simulink model "planmodel_m"  (R2025b)
settings: Solver=ode4  StartTime=0.0  StopTime=200  FixedStep=0.001  RelTol=1e-3
values from neighbouring files (symbols this model uses):
  a0 = 340.294    [plan.m]    (also in plan.mat)
  b_ref = 2.0    (= 2)    [plan.m]    (also in plan.mat)
  c_gear = [0.8e4, 1.4e4, 1.4e4]    [plan.m]    (also in plan.mat = [8000 14000 14000])
  c_lat = [1.4e4, 2.2e4, 2.2e4]    [plan.m]    (also in plan.mat = [14000 22000 22000])
  c_ref = 0.9    [plan.m]    (also in plan.mat)
  c_roll = [0.020, 0.018, 0.018]    [plan.m]    (also in plan.mat = [0.02 0.018 0.018])
  CD0 = 0.045    [plan.m]    (also in plan.mat)
  CL0 = 0.083    [plan.m]    (also in plan.mat)
  CLa = 2.50    (= 2.5)    [plan.m]    (also in plan.mat = 3.8)
  Clb = -0.08    [plan.m]    (also in plan.mat)
  Clda = 0.20    (= 0.2)    [plan.m]    (also in plan.mat = -0.2)
  CLde = 0.25    [plan.m]    (also in plan.mat = 0.28)
  Clp = -0.70    (= -0.7)    [plan.m]    (also in plan.mat)
  CLq = 3.00    (= 3)    [plan.m]    (also in plan.mat = 4.5)
  Clr = 0    [plan.m]    (also in plan.mat = 0.08)
  Cm0 = 0.112    [plan.m]    (also in plan.mat = 0.06)
  Cma = -0.8    [plan.m]    (also in plan.mat)
  Cmde = 0.90    (= 0.9)    [plan.m]    (also in plan.mat = -0.9)
  Cmq = -18.0    (= -18)    [plan.m]    (also in plan.mat)
  Cnb = -0.25    [plan.m]    (also in plan.mat = 0.25)
  Cndr = 0.15    [plan.m]    (also in plan.mat = -0.15)
  Cnp = 0    [plan.m]    (also in plan.mat = -0.04)
  Cnr = -0.45    [plan.m]    (also in plan.mat)
  CSb = -0.8    [plan.m]    (also in plan.mat = -0.7)
  CSdr = 0.18    [plan.m]    (also in plan.mat)
  CSr = 0.15    [plan.m]    (also in plan.mat = 0.12)
  D0 = 800    [plan.m]    (also in plan.mat)
  da_max = 25    [plan.m]    (also in plan.mat)
  da_min = -da_max    (= -25)    [plan.m]    (also in plan.mat)
  de_max = 25    [plan.m]    (also in plan.mat)
  de_min = -de_max    (= -25)    [plan.m]    (also in plan.mat)
  DH = pi / 180    (= 0.0174532925199)    [plan.m]    (also in plan.mat)
  dr_max = 25    [plan.m]    (also in plan.mat)
  dr_min = -dr_max    (= -25)    [plan.m]    (also in plan.mat)
  g = 9.80665    [plan.m]    (also in plan.mat)
  gamma0 = 0.0    (= 0)    [plan.m]
  ground_y = 0.0    (= 0)    [plan.m]
  HD = 180 / pi    (= 57.2957795131)    [plan.m]    (also in plan.mat)
  Ixx = 120.0    (= 120)    [plan.m]    (also in plan.mat)
  Iyy = 480.0    (= 480)    [plan.m]    (also in plan.mat)
  Izz = 520.0    (= 520)    [plan.m]    (also in plan.mat)
  K = 0.080    (= 0.08)    [plan.m]    (also in plan.mat = 0.12)
  K_alpha = 7.67884615385    [plan.mat]
  k_gear = [1.0e5, 3.0e5, 3.0e5]    [plan.m]    (also in plan.mat = [100000 300000 300000])
  k_theta0 = 0.0    (= 0)    [plan.m]
  Kb_to_wy = 10.6510416667    [plan.mat]
  Kn_pitch = 0.117046638908    [plan.mat]
  Kn_to_beta = 0.461367696223    [plan.mat]
  Kw_pitch = -0.524061476442    [plan.mat]
  Kw_to_dr = -1.30612244898    [plan.mat]
  m = 600.0    (= 600)    [plan.m]    (also in plan.mat)
  mu_brake = [0.0, 0.55, 0.55]    [plan.m]    (also in plan.mat = [0 0.55 0.55])
  omigax0 = 0    [plan.m]
  omigay0 = 0    [plan.m]
  omigaz0 = 0    [plan.m]
  psi0 = 0.3/57.3    (= 0.00523560209424)    [plan.m]    (also in plan.mat = 0)
  r_left_b = r_gear_b(:,2)    [plan.m]    (also in plan.mat = [-0.333333333333 -0.8 0.65])
  r_nose_b = r_gear_b(:,1)    [plan.m]    (also in plan.mat = [2 0 0.65])
  r_right_b = r_gear_b(:,3)    [plan.m]    (also in plan.mat = [-0.333333333333 0.8 0.65])
  rho0 = 1.225    [plan.m]    (also in plan.mat)
  S_ref = 1.2    [plan.m]    (also in plan.mat)
  v_eps = 0.20    (= 0.2)    [plan.m]    (also in plan.mat)
  V_min = 1    [plan.m]    (also in plan.mat = 3)
  V_test = 200    [plan.mat]
  Vx0_b = 0.0    (= 0)    [plan.m]
  Vy0_b = 0.0    (= 0)    [plan.m]
  Vz0_b = 0.0    (= 0)    [plan.m]
  W_g = [0; 0; 1]    [plan.m]
  wheel_radius = 0.18    [plan.m]    (also in plan.mat)
  WOW_on = 0.000    (= 0)    [plan.m]    (also in plan.mat)
  Xg0 = 0.0    (= 0)    [plan.m]    (also in plan.mat)
  Yg0 = ground_y + wheel_radius - r_gear_b(2,1) - static_deflection    [plan.m]    (also in plan.mat = 0)
  Zg0 = 1.0    (= 1)    [plan.m]    (also in plan.mat = -0.8215943)
libraries: matrix_library x18, slpidlib x1
(part 2 of 3)

== system planmodel_m/6DOF-MODEL/动力学/体系旋转角速度 ==
  MX : Inport
  MY : Inport  Port=2
  MZ : Inport  Port=3
  Add : Sum
  Add1 : Sum
  Add2 : Sum
  Demux : Demux  Outputs=3
  MATLAB Function : MATLAB Function  TreatAsAtomicUnit=on
  Matrix Multiply1 : Product  Multiplication=Matrix(*)
  Mux : Mux  Inputs=3
  Selector : Selector  InputPortWidth=3  IndexOptions=Index vector (dialog)  Indices=1  OutputSizes=1
  Selector1 : Selector  InputPortWidth=3  IndexOptions=Index vector (dialog)  Indices=2  OutputSizes=1
  Selector2 : Selector  InputPortWidth=3  IndexOptions=Index vector (dialog)  Indices=3  OutputSizes=1
  Subsystem : Subsystem
  Subsystem1 : Subsystem
  Subsystem2 : Subsystem
  wx1 : Outport
  wy1 : Outport  Port=2
  wz1 : Outport  Port=3
  wires:
  Subsystem/1(wx1) -> Subsystem2/2(wx1), Subsystem1/2(wx1), wx1/1
  Subsystem1/1(wy1) -> wy1/1, Subsystem2/3(wy1), Subsystem/3(wy1)
  Subsystem2/1(wz1) -> wz1/1, Subsystem1/3(wz1), Subsystem/2(wz1)
  [M_gear] -> Selector2/1, Selector1/1, Selector/1
  MX/1 -> Add/1
  MY/1 -> Add1/1
  MZ/1 -> Add2/1
  Selector/1 -> Add/2
  Selector2/1 -> Add2/2
  Selector1/1 -> Add1/2
  MATLAB Function/1(R_wind_b) -> Matrix Multiply1/1
  [alpha] -> MATLAB Function/1(alpha)
  [beta] -> MATLAB Function/2(beta)
  Add/1 -> Mux/1
  Add1/1 -> Mux/2
  Add2/1 -> Mux/3
  Mux/1 -> Matrix Multiply1/2
  Demux/1 -> Subsystem/1(MX)
  Matrix Multiply1/1 -> Demux/1
  Demux/2 -> Subsystem1/1(MY)
  Demux/3 -> Subsystem2/1(MZ)

== system planmodel_m/6DOF-MODEL/动力学/姿态角 ==
  wx1 : Inport
  wy1 : Inport  Port=2
  wz1 : Inport  Port=3
  Subsystem : Subsystem
  Subsystem1 : Subsystem
  Subsystem2 : Subsystem
  gamma(eular) : Outport
  theta(eular) : Outport  Port=2
  psi(eular) : Outport  Port=3
  tag scope: gamma_eular=global, psi_eular=global, theta_eular=global
  wires:
  wy1/1 -> Subsystem/2(wy1), Subsystem1/1(wy1), Subsystem2/1(wy1)
  wx1/1 -> Subsystem/1(wx1)
  Subsystem/1(gamma(eular)) -> [gamma_eular], gamma(eular)/1
  wz1/1 -> Subsystem1/2(wz1), Subsystem/3(wz1), Subsystem2/2(wz1)
  Subsystem1/1(theta(eular)) -> [theta_eular], theta(eular)/1
  Subsystem2/1(psi(eular)) -> psi(eular)/1, [psi_eular]

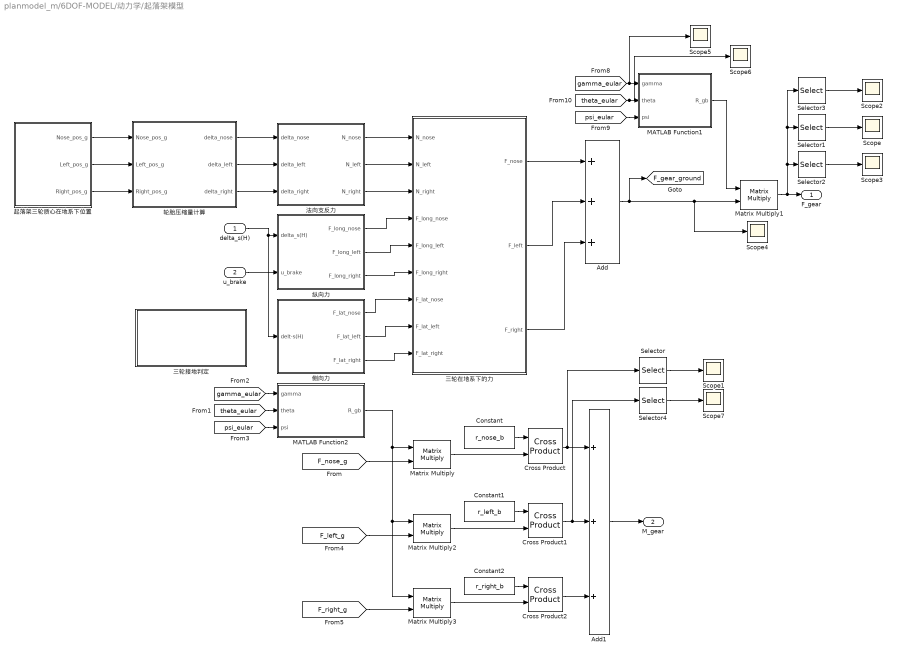
== system planmodel_m/6DOF-MODEL/动力学/起落架模型 ==
  delta_s(H) : Inport
  u_brake : Inport  Port=2
  Add : Sum  Inputs=+++
  Add1 : Sum  Inputs=+++
  Constant : Constant  Value=r_nose_b
  Constant1 : Constant  Value=r_left_b
  Constant2 : Constant  Value=r_right_b
  Cross Product : matrix_library/Cross Product
  Cross Product1 : matrix_library/Cross Product
  Cross Product2 : matrix_library/Cross Product
  MATLAB Function1 : MATLAB Function  TreatAsAtomicUnit=on
  MATLAB Function2 : MATLAB Function  TreatAsAtomicUnit=on
  Matrix Multiply{,1..3} (4 alike) : Product  Multiplication=Matrix(*)
  Scope{,1..7} (8 alike) : Scope
      Scope settings: ActiveDisplayYMinimum=-735.6131  ActiveDisplayYMaximum=6620.5176  DataLoggingVariableName=ScopeData10
      Scope1 settings: ActiveDisplayYMinimum=-1  ActiveDisplayYMaximum=1  DataLoggingVariableName=ScopeData24
      Scope2 settings: ActiveDisplayYMinimum=-144.4872  ActiveDisplayYMaximum=214.9634
      Scope3 settings: ActiveDisplayYMinimum=-1  ActiveDisplayYMaximum=1  DataLoggingVariableName=ScopeData2
      Scope4 settings: ActiveDisplayYMinimum=-856.7234  ActiveDisplayYMaximum=6633.9745  DataLoggingVariableName=ScopeData3
      Scope5 settings: ActiveDisplayYMinimum=1E-13  ActiveDisplayYMaximum=2.6E-13  DataLoggingVariableName=ScopeData4
      Scope6 settings: ActiveDisplayYMinimum=-2E-18  ActiveDisplayYMaximum=3.3E-17  DataLoggingVariableName=ScopeData5
      Scope7 settings: ActiveDisplayYMinimum=-1  ActiveDisplayYMaximum=1  DataLoggingVariableName=ScopeData4
  Selector : Selector  InputPortWidth=3  IndexOptions=Index vector (dialog)  Indices=3  OutputSizes=1
  Selector1 : Selector  InputPortWidth=3  IndexOptions=Index vector (dialog)  Indices=2  OutputSizes=1
  Selector2 : Selector  InputPortWidth=3  IndexOptions=Index vector (dialog)  Indices=3  OutputSizes=1
  Selector3 : Selector  InputPortWidth=3  IndexOptions=Index vector (dialog)  Indices=1  OutputSizes=1
  Selector4 : Selector  InputPortWidth=3  IndexOptions=Index vector (dialog)  Indices=3  OutputSizes=1
  三轮在地系下的力 : Subsystem
  三轮接地判定 : Subsystem
  侧向力 : Subsystem
  法向支反力 : Subsystem
  纵向力 : Subsystem
  起落架三轮质心在地系下位置 : Subsystem
  轮胎压缩量计算 : Subsystem
  F_gear : Outport
  M_gear : Outport  Port=2
  tag scope: F_gear_ground=global
  wires:
  起落架三轮质心在地系下位置/1(Nose_pos_g) -> 轮胎压缩量计算/1(Nose_pos_g)
  起落架三轮质心在地系下位置/2(Left_pos_g) -> 轮胎压缩量计算/2(Left_pos_g)
  起落架三轮质心在地系下位置/3(Right_pos_g) -> 轮胎压缩量计算/3(Right_pos_g)
  轮胎压缩量计算/1(delta_nose) -> 法向支反力/1(delta_nose)
  轮胎压缩量计算/2(delta_left) -> 法向支反力/2(delta_left)
  轮胎压缩量计算/3(delta_right) -> 法向支反力/3(delta_right)
  delta_s(H)/1 -> 侧向力/1(delt-s(H)), 纵向力/1(delta_s(H))
  u_brake/1 -> 纵向力/2(u_brake)
  法向支反力/1(N_nose) -> 三轮在地系下的力/1(N_nose)
  法向支反力/2(N_left) -> 三轮在地系下的力/2(N_left)
  法向支反力/3(N_right) -> 三轮在地系下的力/3(N_right)
  纵向力/1(F_long_nose) -> 三轮在地系下的力/4(F_long_nose)
  纵向力/2(F_long_left) -> 三轮在地系下的力/5(F_long_left)
  纵向力/3(F_long_right) -> 三轮在地系下的力/6(F_long_right)
  侧向力/1(F_lat_nose) -> 三轮在地系下的力/7(F_lat_nose)
  侧向力/2(F_lat_left) -> 三轮在地系下的力/8(F_lat_left)
  侧向力/3(F_lat_right) -> 三轮在地系下的力/9(F_lat_right)
  三轮在地系下的力/1(F_nose) -> Add/1
  三轮在地系下的力/2(F_left) -> Add/2
  三轮在地系下的力/3(F_right) -> Add/3
  Add/1 -> Scope4/1, Matrix Multiply1/2, [F_gear_ground]
  MATLAB Function1/1(R_gb) -> Matrix Multiply1/1
  [gamma_eular] -> Scope5/1, MATLAB Function1/1(gamma)
  Matrix Multiply1/1 -> Selector3/1, Selector1/1, Selector2/1, F_gear/1
  Constant/1 -> Cross Product/1
  Constant1/1 -> Cross Product1/1
  Constant2/1 -> Cross Product2/1
  Cross Product/1 -> Add1/1, Selector/1
  Cross Product1/1 -> Selector4/1, Add1/2
  Cross Product2/1 -> Add1/3
  Add1/1 -> M_gear/1
  [theta_eular] -> Scope6/1, MATLAB Function1/2(theta)
  [psi_eular] -> MATLAB Function1/3(psi)
  [theta_eular] -> MATLAB Function2/2(theta)
  [gamma_eular] -> MATLAB Function2/1(gamma)
  [psi_eular] -> MATLAB Function2/3(psi)
  MATLAB Function2/1(R_gb) -> Matrix Multiply3/1, Matrix Multiply2/1, Matrix Multiply/1
  [F_nose_g] -> Matrix Multiply/2
  [F_right_g] -> Matrix Multiply3/2
  [F_left_g] -> Matrix Multiply2/2
  Matrix Multiply2/1 -> Cross Product1/2
  Matrix Multiply3/1 -> Cross Product2/2
  Matrix Multiply/1 -> Cross Product/2
  Selector1/1 -> Scope/1
  Selector3/1 -> Scope2/1
  Selector2/1 -> Scope3/1
  Selector/1 -> Scope1/1
  Selector4/1 -> Scope7/1

== system planmodel_m/control/俯仰通道控制器/俯仰通道 ==
  nyc : Inport
  ny : Inport  Port=2
  wz : Inport  Port=3
  Constant : Constant
  Div : Product  Inputs=/*
  Gain : Gain
  Gain2 : Gain
  Integrator : Integrator  ExternalReset=either  LimitOutput=on  UpperSaturationLimit=5  LowerSaturationLimit=-5
  Ka : Constant  Value=K_alpha
  Kn : Constant  Value=Kn_pitch
  Kwz : Constant  Value=Kw_pitch
  Pk : Product
  Pn : Product
  Product : Product
  Product1 : Product
  Product2 : Product
  Sat : Saturate  UpperLimit=10  LowerLimit=0.25
  Scope : Scope  NumInputPorts=2
      settings: ActiveDisplayYMinimum=0.47912  ActiveDisplayYMaximum=1.5066
  Sqr : Math  Operator=square
  Sum{,1..3} (4 alike) : Sum  Inputs=|+-
  VRef : Constant  Value=V_test
  伪攻角回路 : Subsystem
  delta_e : Outport
  wires:
  Kn/1 -> Product/1
  VRef/1 -> Div/1
  Integrator/1 -> Sum1/1
  [Vg] -> Div/2
  Pk/1 -> delta_e/1
  nyc/1 -> Sum/1, Scope/1
  ny/1 -> Sum/2, Scope/2
  Div/1 -> Sqr/1
  Sqr/1 -> Sat/1
  Sum/1 -> Product/2
  Product/1 -> Pn/1
  Constant/1 -> Sum3/1
  Sat/1 -> Pn/2, Pk/2
  [no_contact] -> Sum3/2
  Kwz/1 -> Gain2/1
  Pn/1 -> Integrator/1
  Sum3/1 -> Integrator/2
  wz/1 -> 伪攻角回路/1(wz), Sum2/2
  Ka/1 -> Gain/1
  伪攻角回路/1(alpha_c) -> Sum1/2
  Gain/1 -> Product1/1
  Sum1/1 -> Product1/2
  Product1/1 -> Sum2/1
  Gain2/1 -> Product2/1
  Sum2/1 -> Product2/2
  Product2/1 -> Pk/1

== system planmodel_m/control/俯仰通道控制器/抬轮俯仰角控制通道 ==
  theta_cmd(H) : Inport
  Gain1 : Gain
  K_theta : Gain  Gain=1.3
  Sum : Sum  Inputs=|+-
  Sum1 : Sum  Inputs=|+-
  de : Outport
  wires:
  theta_cmd(H)/1 -> Sum/1
  [theta_eular] -> Sum/2
  Sum/1 -> K_theta/1
  K_theta/1 -> Sum1/1
  [wz1] -> Gain1/1
  Gain1/1 -> Sum1/2
  Sum1/1 -> de/1

== system planmodel_m/control/滚转通道控制器/Subsystem ==
  gamma_c : Inport
  wx : Inport  Port=2
  gamma : Inport  Port=3
  Gain1 : Gain  Gain=1/HD
  Integrator : Integrator
  Product : Product
  Product1 : Product
  Product2 : Product
  Scope : Scope  NumInputPorts=2
      settings: ActiveDisplayYMinimum=-0.00046391  ActiveDisplayYMaximum=0.00061315  DataLoggingVariableName=ScopeData2
  Scope1 : Scope
      settings: ActiveDisplayYMinimum=-1  ActiveDisplayYMaximum=1  DataLoggingVariableName=ScopeData47
  Sum : Sum  Inputs=|+-
  Sum1 : Sum  Inputs=|+-
  Sum2 : Sum  Inputs=|++
  kgamma_to_wx : Constant  Value=3
  kigamma_to_wx : Constant
  kwx_to_da : Constant  Value=0.5
  da : Outport
  wires:
  Sum/1 -> Product/2, Product2/2
  Sum1/1 -> Product1/2
  wx/1 -> Sum1/2
  gamma/1 -> Scope/2, Sum/2
  kigamma_to_wx/1 -> Product2/1
  Product2/1 -> Integrator/1
  Product/1 -> Sum2/1
  Sum2/1 -> Sum1/1
  Integrator/1 -> Sum2/2
  Gain1/1 -> Scope/1, Sum/1
  kgamma_to_wx/1 -> Product/1
  kwx_to_da/1 -> Product1/1
  gamma_c/1 -> Gain1/1
  Product1/1 -> Scope1/1, da/1

== system planmodel_m/control/航向通道控制器/偏航通道 ==
  nzc : Inport
  nz : Inport  Port=2
  wy : Inport  Port=3
  Constant1 : Constant
  Constant3 : Constant  Value=0
  Div : Product  Inputs=/*
  Gain : Gain  Gain=-Kn_to_beta
  Gain1 : Gain  Gain=Kb_to_wy
  Gain2 : Gain  Gain=Kw_to_dr
  Gain4 : Gain  Gain=HD
  Integrator : Integrator  ExternalReset=either
  Pk : Product
  Pn : Product
  Sat : Saturate  UpperLimit=10  LowerLimit=0.25
  Saturation1 : Saturate  UpperLimit=0.2*57.3  LowerLimit=-0.2*57.3
  Scope : Scope  NumInputPorts=2
      settings: ActiveDisplayYMinimum=-0.21765504645958114  ActiveDisplayYMaximum=0.42871368847964081
  Scope1 : Scope
      settings: ActiveDisplayYMinimum=-0.34545426181804578  ActiveDisplayYMaximum=0.23208089486151426  DataLoggingVariableName=ScopeData42
  Scope12 : Scope
      settings: ActiveDisplayYMinimum=-1.8487  ActiveDisplayYMaximum=16.1209  DataLoggingVariableName=ScopeData39
  Scope2 : Scope  NumInputPorts=2
      settings: ActiveDisplayYMinimum=-1.0707329995063326  ActiveDisplayYMaximum=0.50557097548372176  DataLoggingVariableName=ScopeData41
  Sqr : Math  Operator=square
  Sum : Sum  Inputs=|+-
  Sum1 : Sum  Inputs=|+-
  Sum2 : Sum  Inputs=|+-
  Switch2 : Switch  Threshold=40  SaturateOnIntegerOverflow=off  InputSameDT=off
  VRef : Constant  Value=V_test
  伪攻角回路 : Subsystem
  delta_r : Outport
  wires:
  nz/1 -> Sum/2, Scope/2
  nzc/1 -> Scope/1, Sum/1
  Constant1/1 -> Switch2/1
  Constant3/1 -> Switch2/3
  [Vg] -> Div/2, Switch2/2
  Gain4/1 -> Scope12/1
  [psi_eular] -> Gain4/1
  wy/1 -> Scope2/2, Sum2/2, 伪攻角回路/1(wy)
  伪攻角回路/1(beta_c) -> Sum1/2
  Sum1/1 -> Gain1/1
  Gain1/1 -> Scope2/1, Sum2/1
  Sum2/1 -> Gain2/1
  Sum/1 -> Gain/1
  Integrator/1 -> Saturation1/1
  Saturation1/1 -> Sum1/1
  Switch2/1 -> Integrator/2
  VRef/1 -> Div/1
  Div/1 -> Sqr/1
  Sqr/1 -> Sat/1
  Sat/1 -> Pn/2, Pk/2
  Gain2/1 -> Pk/1
  Pk/1 -> delta_r/1, Scope1/1
  Gain/1 -> Pn/1
  Pn/1 -> Integrator/1

== system planmodel_m/control/航向通道控制器/地面转向控制 ==
  Z_cmd : Inport
  Gain : Gain  Gain=0.8
  Gain4 : Gain  Gain=HD
  K_z : Constant  Value=0.04
  Product : Product
  Saturation1 : Saturate  UpperLimit=5  LowerLimit=-5
  Scope : Scope  NumInputPorts=2
      settings: ActiveDisplayYMinimum=-14.247959246651458  ActiveDisplayYMaximum=14.936251376866672  DataLoggingVariableName=ScopeData26
  Scope12 : Scope
      settings: ActiveDisplayYMinimum=-16.1569  ActiveDisplayYMaximum=26.4194  DataLoggingVariableName=ScopeData32
  Scope25 : Scope
      settings: ActiveDisplayYMinimum=-11.4126  ActiveDisplayYMaximum=3.1927  DataLoggingVariableName=ScopeData31
  Sum : Sum  Inputs=|+-
  Sum1 : Sum  Inputs=|++
  Transfer Fcn : TransferFcn  Denominator=[0.1 1]
  delta_s(H) : Outport
  wires:
  Z_cmd/1 -> Scope/1, Sum/1
  [Z_positon] -> Scope/2, Sum/2
  K_z/1 -> Product/1
  [delta_s] -> Scope25/1
  [psi_eular] -> Gain/1
  Gain4/1 -> Scope12/1
  [psi_eular] -> Gain4/1
  Gain/1 -> Sum1/2
  Sum/1 -> Saturation1/1
  Product/1 -> Sum1/1
  Saturation1/1 -> Product/2
  Sum1/1 -> Transfer Fcn/1
  Transfer Fcn/1 -> delta_s(H)/1

== system planmodel_m/control/航向通道控制器1/偏航通道 ==
  nzc : Inport
  nz : Inport  Port=2
  wy : Inport  Port=3
  Constant1 : Constant
  Constant3 : Constant  Value=0
  Gain : Gain  Gain=-Kn_to_beta
  Gain1 : Gain  Gain=Kb_to_wy
  Gain2 : Gain  Gain=Kw_to_dr
  Gain4 : Gain  Gain=HD
  Integrator : Integrator  ExternalReset=either
  Saturation1 : Saturate  UpperLimit=0.2*57.3  LowerLimit=-0.2*57.3
  Scope : Scope  NumInputPorts=2
      settings: ActiveDisplayYMinimum=-0.48826  ActiveDisplayYMaximum=1.2494
  Scope1 : Scope
      settings: ActiveDisplayYMinimum=-153.0484  ActiveDisplayYMaximum=1377.4356  DataLoggingVariableName=ScopeData42
  Scope12 : Scope
      settings: ActiveDisplayYMinimum=-151.9167  ActiveDisplayYMaximum=542.4127  DataLoggingVariableName=ScopeData39
  Scope2 : Scope  NumInputPorts=2
      settings: ActiveDisplayYMinimum=-6.2342  ActiveDisplayYMaximum=4.3442  DataLoggingVariableName=ScopeData41
  Sum : Sum  Inputs=|+-
  Sum1 : Sum  Inputs=|+-
  Sum2 : Sum  Inputs=|+-
  Switch2 : Switch  Threshold=40  SaturateOnIntegerOverflow=off  InputSameDT=off
  伪攻角回路 : Subsystem
  delta_r : Outport
  wires:
  nz/1 -> Scope/2, Sum/2
  nzc/1 -> Scope/1, Sum/1
  Constant1/1 -> Switch2/1
  Constant3/1 -> Switch2/3
  [Vg] -> Switch2/2
  Gain4/1 -> Scope12/1
  [psi_eular] -> Gain4/1
  wy/1 -> Scope2/2, Sum2/2, 伪攻角回路/1(wy)
  伪攻角回路/1(beta_c) -> Sum1/2
  Sum1/1 -> Gain1/1
  Gain1/1 -> Scope2/1, Sum2/1
  Sum2/1 -> Gain2/1
  Gain2/1 -> Scope1/1, delta_r/1
  Gain/1 -> Integrator/1
  Sum/1 -> Gain/1
  Integrator/1 -> Saturation1/1
  Saturation1/1 -> Sum1/1
  Switch2/1 -> Integrator/2

== system planmodel_m/control/航向通道控制器1/地面转向控制 ==
  Z_cmd : Inport
  Gain : Gain  Gain=0.8
  Gain4 : Gain  Gain=HD
  K_z : Constant  Value=0.04
  Product : Product
  Saturation1 : Saturate  UpperLimit=5  LowerLimit=-5
  Scope : Scope  NumInputPorts=2
      settings: ActiveDisplayYMinimum=-8.5383  ActiveDisplayYMaximum=8.0262  DataLoggingVariableName=ScopeData26
  Scope12 : Scope
      settings: ActiveDisplayYMinimum=-4.9887  ActiveDisplayYMaximum=24.3498  DataLoggingVariableName=ScopeData32
  Scope25 : Scope
      settings: ActiveDisplayYMinimum=-13.1282  ActiveDisplayYMaximum=3.562  DataLoggingVariableName=ScopeData31
  Sum : Sum  Inputs=|+-
  Sum1 : Sum  Inputs=|++
  delta_s(H) : Outport
  wires:
  Z_cmd/1 -> Scope/1, Sum/1
  [Z_positon] -> Scope/2, Sum/2
  K_z/1 -> Product/1
  [delta_s] -> Scope25/1
  [psi_eular] -> Gain/1
  Gain4/1 -> Scope12/1
  [psi_eular] -> Gain4/1
  Gain/1 -> Sum1/2
  Sum/1 -> Saturation1/1
  Product/1 -> Sum1/1
  Saturation1/1 -> Product/2
  Sum1/1 -> delta_s(H)/1

== system planmodel_m/6DOF-MODEL/AERO-PARAMETER/无量纲化角速率/Subsystem ==
  wy1 : Inport
  Va : Inport  Port=2
  Constant4 : Constant  Value=b_ref
  Divide : Product  Inputs=*/
  Gain : Gain  Gain=2
  Product : Product
  r_hat : Outport
  wires:
  Va/1 -> Gain/1
  wy1/1 -> Product/1
  Constant4/1 -> Product/2
  Product/1 -> Divide/1
  Divide/1 -> r_hat/1
  Gain/1 -> Divide/2

== system planmodel_m/6DOF-MODEL/AERO-PARAMETER/无量纲化角速率/Subsystem1 ==
  wz1 : Inport
  Va : Inport  Port=2
  Constant4 : Constant  Value=c_ref
  Divide : Product  Inputs=*/
  Gain : Gain  Gain=2
  Product : Product
  Scope : Scope
      settings: ActiveDisplayYMinimum=-0.31338  ActiveDisplayYMaximum=0.53416  DataLoggingVariableName=ScopeData22
  q_hat : Outport
  wires:
  Va/1 -> Gain/1
  wz1/1 -> Scope/1, Product/1
  Constant4/1 -> Product/2
  Product/1 -> Divide/1
  Divide/1 -> q_hat/1
  Gain/1 -> Divide/2

== system planmodel_m/6DOF-MODEL/AERO-PARAMETER/无量纲化角速率/Subsystem2 ==
  wx1 : Inport
  Va : Inport  Port=2
  Constant4 : Constant  Value=b_ref
  Divide : Product  Inputs=*/
  Gain : Gain  Gain=2
  Product : Product
  p_hat : Outport
  wires:
  Va/1 -> Gain/1
  wx1/1 -> Product/1
  Constant4/1 -> Product/2
  Product/1 -> Divide/1
  Divide/1 -> p_hat/1
  Gain/1 -> Divide/2

== system planmodel_m/6DOF-MODEL/动力学/Subsystem3/WindCorrection ==
  vx1 : Inport
  vy1 : Inport  Port=2
  vz1 : Inport  Port=3
  W_g : Constant  Value=W_g
  wind_calc : MATLAB Function  TreatAsAtomicUnit=on
  vx1_air : Outport
  vy1_air : Outport  Port=2
  vz1_air : Outport  Port=3
  wires:
  wind_calc/3(vz_air) -> vz1_air/1
  wind_calc/1(vx_air) -> vx1_air/1
  vx1/1 -> wind_calc/1(vx)
  W_g/1 -> wind_calc/5(W_g)
  vy1/1 -> wind_calc/2(vy)
  vz1/1 -> wind_calc/3(vz)
  [Tbg] -> wind_calc/4(R_gb)
  wind_calc/2(vy_air) -> vy1_air/1

== system planmodel_m/6DOF-MODEL/动力学/v在体系下的分量/Subsystem ==
  Fx/m : Inport
  wy1 : Inport  Port=2
  wz1 : Inport  Port=3
  vz : Inport  Port=4
  vy : Inport  Port=5
  Product1 : Product
  Product4 : Product
  Subtract1 : Sum  Inputs=+-
  Subtract3 : Sum  Inputs=+-
  vx_dot : Outport
  wires:
  Fx/m/1 -> Subtract3/1
  Subtract3/1 -> vx_dot/1
  Subtract1/1 -> Subtract3/2
  vy/1 -> Product4/2
  wz1/1 -> Product4/1
  Product4/1 -> Subtract1/2
  wy1/1 -> Product1/1
  vz/1 -> Product1/2
  Product1/1 -> Subtract1/1

== system planmodel_m/6DOF-MODEL/动力学/v在体系下的分量/Subsystem1 ==
  Fy/m : Inport
  wx1 : Inport  Port=2
  wz1 : Inport  Port=3
  vx : Inport  Port=4
  vz : Inport  Port=5
  Product1 : Product
  Product4 : Product
  Subtract2 : Sum  Inputs=+-
  Subtract3 : Sum  Inputs=+-
  vy_dot : Outport
  wires:
  Fy/m/1 -> Subtract3/1
  Subtract3/1 -> vy_dot/1
  vx/1 -> Product4/1
  wz1/1 -> Product4/2
  wx1/1 -> Product1/1
  vz/1 -> Product1/2
  Product4/1 -> Subtract2/1
  Product1/1 -> Subtract2/2
  Subtract2/1 -> Subtract3/2

== system planmodel_m/6DOF-MODEL/动力学/v在体系下的分量/Subsystem2 ==
  Fz/m : Inport
  wx1 : Inport  Port=2
  wy1 : Inport  Port=3
  vx : Inport  Port=4
  vy : Inport  Port=5
  Product1 : Product
  Product2 : Product
  Subtract2 : Sum  Inputs=+-
  Subtract3 : Sum  Inputs=+-
  vz_dot : Outport
  wires:
  Fz/m/1 -> Subtract3/1
  Subtract3/1 -> vz_dot/1
  Subtract2/1 -> Subtract3/2
  Product1/1 -> Subtract2/1
  wx1/1 -> Product1/1
  vy/1 -> Product1/2
  wy1/1 -> Product2/1
  vx/1 -> Product2/2
  Product2/1 -> Subtract2/2

== system planmodel_m/6DOF-MODEL/动力学/体系旋转角速度/Subsystem ==
  MX : Inport
  wz1 : Inport  Port=2
  wy1 : Inport  Port=3
  Constant : Constant  Value=Ixx
  Constant1 : Constant  Value=Izz
  Constant2 : Constant  Value=Iyy
  Divide : Product  Inputs=*/
  Integrator : Integrator  InitialCondition=omigax0
  Product : Product
  Product1 : Product
  Subtract : Sum  Inputs=+-
  Sum : Sum  Inputs=|+-
  wx1 : Outport
  wires:
  MX/1 -> Sum/1
  Sum/1 -> Divide/1
  Constant/1 -> Divide/2
  Subtract/1 -> Product/1
  wz1/1 -> Product1/1
  wy1/1 -> Product1/2
  Product1/1 -> Product/2
  Constant1/1 -> Subtract/1
  Constant2/1 -> Subtract/2
  Product/1 -> Sum/2
  Divide/1 -> Integrator/1
  Integrator/1 -> wx1/1

== system planmodel_m/6DOF-MODEL/动力学/体系旋转角速度/Subsystem1 ==
  MY : Inport
  wx1 : Inport  Port=2
  wz1 : Inport  Port=3
  Constant : Constant  Value=Iyy
  Constant1 : Constant  Value=Ixx
  Constant2 : Constant  Value=Izz
  Divide : Product  Inputs=*/
  Integrator : Integrator  InitialCondition=omigay0
  Product : Product
  Product1 : Product
  Subtract : Sum  Inputs=+-
  Sum : Sum  Inputs=|+-
  wy1 : Outport
  wires:
  MY/1 -> Sum/1
  Sum/1 -> Divide/1
  Constant/1 -> Divide/2
  Subtract/1 -> Product/1
  wx1/1 -> Product1/1
  wz1/1 -> Product1/2
  Product1/1 -> Product/2
  Constant1/1 -> Subtract/1
  Constant2/1 -> Subtract/2
  Product/1 -> Sum/2
  Divide/1 -> Integrator/1
  Integrator/1 -> wy1/1

== system planmodel_m/6DOF-MODEL/动力学/体系旋转角速度/Subsystem2 ==
  MZ : Inport
  wx1 : Inport  Port=2
  wy1 : Inport  Port=3
  Constant : Constant  Value=Izz
  Constant1 : Constant  Value=Iyy
  Constant2 : Constant  Value=Ixx
  Divide : Product  Inputs=*/
  Integrator : Integrator  InitialCondition=omigaz0
  Product : Product
  Product1 : Product
  Subtract : Sum  Inputs=+-
  Sum : Sum  Inputs=|+-
  wz1 : Outport
  wires:
  MZ/1 -> Sum/1
  Sum/1 -> Divide/1
  Constant/1 -> Divide/2
  Subtract/1 -> Product/1
  wx1/1 -> Product1/1
  wy1/1 -> Product1/2
  Product1/1 -> Product/2
  Constant1/1 -> Subtract/1
  Constant2/1 -> Subtract/2
  Product/1 -> Sum/2
  Divide/1 -> Integrator/1
  Integrator/1 -> wz1/1

== system planmodel_m/6DOF-MODEL/动力学/姿态角/Subsystem ==
  wx1 : Inport
  wy1 : Inport  Port=2
  wz1 : Inport  Port=3
  Integrator : Integrator  InitialCondition=gamma0
  Product : Product
  Product1 : Product
  Product2 : Product
  Subtract : Sum  Inputs=+-
  Sum : Sum  Inputs=|+-
  Trigonometric Function1 : Trigonometry  Operator=cos
  Trigonometric Function2 : Trigonometry
  Trigonometric Function8 : Trigonometry  Operator=tan
  gamma(eular) : Outport
  wires:
  wx1/1 -> Sum/1
  [gamma_eular] -> Trigonometric Function2/1, Trigonometric Function1/1
  Trigonometric Function1/1 -> Product/2
  wy1/1 -> Product/1
  Trigonometric Function2/1 -> Product1/1
  wz1/1 -> Product1/2
  Product/1 -> Subtract/1
  Product1/1 -> Subtract/2
  Subtract/1 -> Product2/2
  [theta_eular] -> Trigonometric Function8/1
  Trigonometric Function8/1 -> Product2/1
  Sum/1 -> Integrator/1
  Integrator/1 -> gamma(eular)/1
  Product2/1 -> Sum/2

== system planmodel_m/6DOF-MODEL/动力学/姿态角/Subsystem1 ==
  wy1 : Inport
  wz1 : Inport  Port=2
  Integrator : Integrator  InitialCondition=k_theta0
  Product : Product
  Product1 : Product
  Subtract : Sum
  Trigonometric Function1 : Trigonometry
  Trigonometric Function2 : Trigonometry  Operator=cos
  theta(eular) : Outport
  wires:
  [gamma_eular] -> Trigonometric Function2/1, Trigonometric Function1/1
  Trigonometric Function1/1 -> Product/2
  wy1/1 -> Product/1
  Trigonometric Function2/1 -> Product1/1
  wz1/1 -> Product1/2
  Product/1 -> Subtract/1
  Product1/1 -> Subtract/2
  Subtract/1 -> Integrator/1
  Integrator/1 -> theta(eular)/1

== system planmodel_m/6DOF-MODEL/动力学/姿态角/Subsystem2 ==
  wy1 : Inport
  wz1 : Inport  Port=2
  Divide : Product  Inputs=*/
  Integrator : Integrator  InitialCondition=psi0
  Product : Product
  Product1 : Product
  Subtract : Sum  Inputs=+-
  Trigonometric Function1 : Trigonometry  Operator=cos
  Trigonometric Function2 : Trigonometry
  Trigonometric Function8 : Trigonometry  Operator=cos
  psi(eular) : Outport
  wires:
  [gamma_eular] -> Trigonometric Function2/1, Trigonometric Function1/1
  Trigonometric Function1/1 -> Product/2
  wy1/1 -> Product/1
  Trigonometric Function2/1 -> Product1/1
  wz1/1 -> Product1/2
  Product/1 -> Subtract/1
  Product1/1 -> Subtract/2
  [theta_eular] -> Trigonometric Function8/1
  Integrator/1 -> psi(eular)/1
  Subtract/1 -> Divide/1
  Trigonometric Function8/1 -> Divide/2
  Divide/1 -> Integrator/1

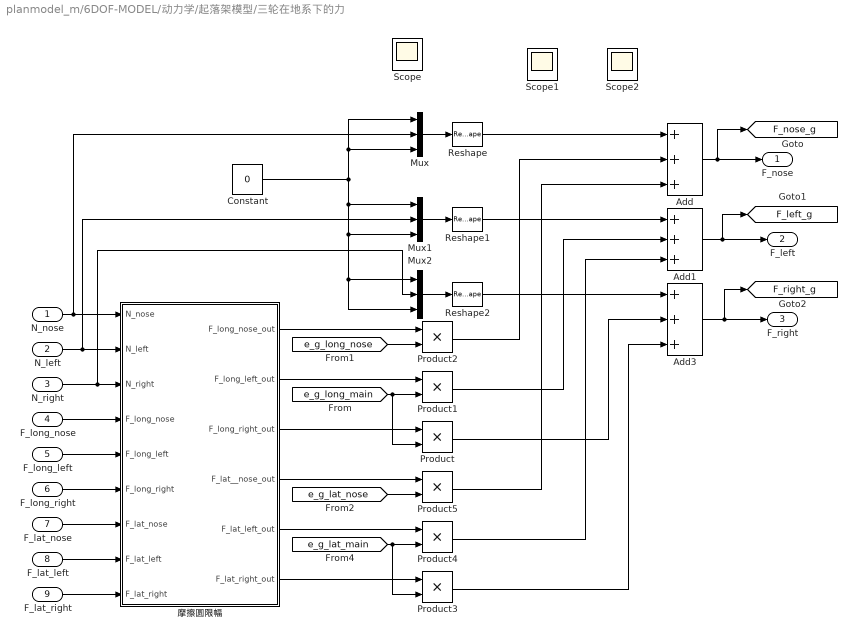
== system planmodel_m/6DOF-MODEL/动力学/起落架模型/三轮在地系下的力 ==
  N_nose : Inport
  N_left : Inport  Port=2
  N_right : Inport  Port=3
  F_long_nose : Inport  Port=4
  F_long_left : Inport  Port=5
  F_long_right : Inport  Port=6
  F_lat_nose : Inport  Port=7
  F_lat_left : Inport  Port=8
  F_lat_right : Inport  Port=9
  Add : Sum  Inputs=+++
  Add1 : Sum  Inputs=+++
  Add3 : Sum  Inputs=+++
  Constant : Constant  Value=0
  Mux : Mux  Inputs=3
  Mux1 : Mux  Inputs=3
  Mux2 : Mux  Inputs=3
  Product{,1..5} (6 alike) : Product
  Reshape : Reshape  OutputDimensionality=Column vector (2-D)
  Reshape1 : Reshape  OutputDimensionality=Column vector (2-D)
  Reshape2 : Reshape  OutputDimensionality=Column vector (2-D)
  Scope : Scope
      settings: ActiveDisplayYMinimum=-1  ActiveDisplayYMaximum=1  DataLoggingVariableName=ScopeData12
  Scope1 : Scope
      settings: ActiveDisplayYMinimum=-3888.8593  ActiveDisplayYMaximum=34999.7335  DataLoggingVariableName=ScopeData13
  Scope2 : Scope
      settings: ActiveDisplayYMinimum=-1  ActiveDisplayYMaximum=1  DataLoggingVariableName=ScopeData14
  摩擦圆限幅 : Subsystem
  F_nose : Outport
  F_left : Outport  Port=2
  F_right : Outport  Port=3
  tag scope: F_left_g=global, F_nose_g=global, F_right_g=global
  wires:
  Product1/1 -> Add1/2
  Constant/1 -> Mux2/3, Mux2/1, Mux1/3, Mux1/1, Mux/1, Mux/3
  [e_g_long_nose] -> Product2/2
  [e_g_long_main] -> Product/2, Product1/2
  Product5/1 -> Add/3
  Product2/1 -> Add/2
  Product/1 -> Add3/2
  [e_g_lat_nose] -> Product5/2
  [e_g_lat_main] -> Product3/2, Product4/2
  Product4/1 -> Add1/3
  Product3/1 -> Add3/3
  Add/1 -> [F_nose_g], F_nose/1
  Add1/1 -> [F_left_g], F_left/1
  Add3/1 -> [F_right_g], F_right/1
  Mux/1 -> Reshape/1
  Mux2/1 -> Reshape2/1
  Reshape2/1 -> Add3/1
  Reshape1/1 -> Add1/1
  Mux1/1 -> Reshape1/1
  Reshape/1 -> Add/1
  N_nose/1 -> Mux/2, 摩擦圆限幅/1(N_nose)
  N_left/1 -> Mux1/2, 摩擦圆限幅/2(N_left)
  N_right/1 -> Mux2/2, 摩擦圆限幅/3(N_right)
  F_long_nose/1 -> 摩擦圆限幅/4(F_long_nose)
  F_long_left/1 -> 摩擦圆限幅/5(F_long_left)
  F_long_right/1 -> 摩擦圆限幅/6(F_long_right)
  F_lat_nose/1 -> 摩擦圆限幅/7(F_lat_nose)
  F_lat_left/1 -> 摩擦圆限幅/8(F_lat_left)
  F_lat_right/1 -> 摩擦圆限幅/9(F_lat_right)
  摩擦圆限幅/1(F_long_nose_out) -> Product2/1
  摩擦圆限幅/4(F_lat__nose_out) -> Product5/1
  摩擦圆限幅/2(F_long_left_out) -> Product1/1
  摩擦圆限幅/5(F_lat_left_out) -> Product4/1
  摩擦圆限幅/3(F_long_right_out) -> Product/1
  摩擦圆限幅/6(F_lat_right_out) -> Product3/1

== system planmodel_m/6DOF-MODEL/动力学/起落架模型/三轮接地判定 ==
  Logical Operator : Logic  AllPortsSameDT=off  OutDataTypeStr=boolean
  Logical Operator1 : Logic  Operator=NOR  Inputs=3  AllPortsSameDT=off  OutDataTypeStr=boolean
  tag scope: contact_main=global, no_contact=global
  wires:
  Logical Operator/1 -> [contact_main]
  [contact_nose] -> Logical Operator1/1
  [contact_left] -> Logical Operator1/2, Logical Operator/1
  [contact_right] -> Logical Operator1/3, Logical Operator/2
  Logical Operator1/1 -> [no_contact]

== system planmodel_m/6DOF-MODEL/动力学/起落架模型/侧向力 ==
  delt-s(H) : Inport
  Constant : Constant  Value=c_lat
  Demux : Demux  Outputs=3
  Gain : Gain  Gain=-1
  Gain1 : Gain  Gain=-1
  Gain2 : Gain  Gain=-1
  Product : Product
  Product1 : Product
  Product2 : Product
  Subsystem : Subsystem
  Subsystem1 : Subsystem
  Subsystem2 : Subsystem
  Subsystem3 : Subsystem
  F_lat_nose : Outport
  F_lat_left : Outport  Port=2
  F_lat_right : Outport  Port=3
  wires:
  delt-s(H)/1 -> Subsystem/1(delt-s(H))
  Constant/1 -> Demux/1
  Subsystem/1(V_lat_nose) -> Product/1
  Demux/1 -> Product/2
  Subsystem/2(V_lat_left) -> Product1/1
  Subsystem/3(V_lat_right) -> Product2/1
  Demux/2 -> Product1/2
  Demux/3 -> Product2/2
  Product/1 -> Gain/1
  Product1/1 -> Gain1/1
  Product2/1 -> Gain2/1
  Gain/1 -> Subsystem2/1(In1)
  Subsystem2/1(F_lat_nose) -> F_lat_nose/1
  Gain1/1 -> Subsystem1/1(In1)
  Subsystem1/1(F_lat_left) -> F_lat_left/1
  Gain2/1 -> Subsystem3/1(In1)
  Subsystem3/1(F_lat_right) -> F_lat_right/1

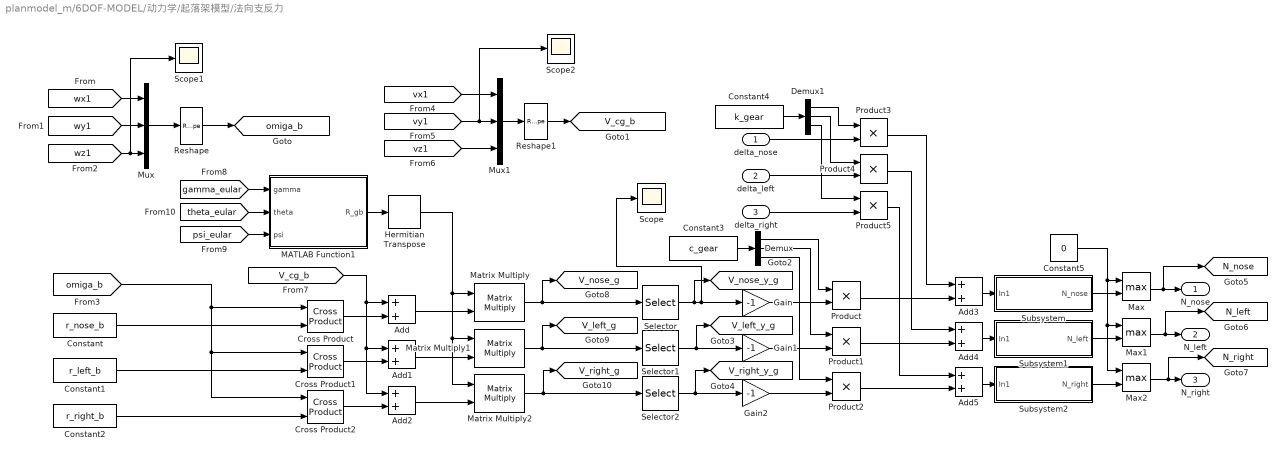
== system planmodel_m/6DOF-MODEL/动力学/起落架模型/法向支反力 ==
  delta_nose : Inport
  delta_left : Inport  Port=2
  delta_right : Inport  Port=3
  Add{,1..5} (6 alike) : Sum
  Constant : Constant  Value=r_nose_b
  Constant1 : Constant  Value=r_left_b
  Constant2 : Constant  Value=r_right_b
  Constant3 : Constant  Value=c_gear
  Constant4 : Constant  Value=k_gear
  Constant5 : Constant  Value=0
  Cross Product : matrix_library/Cross Product
  Cross Product1 : matrix_library/Cross Product
  Cross Product2 : matrix_library/Cross Product
  Demux : Demux  Outputs=3
  Demux1 : Demux  Outputs=3
  Gain : Gain  Gain=-1
  Gain1 : Gain  Gain=-1
  Gain2 : Gain  Gain=-1
  Hermitian Transpose : matrix_library/Hermitian Transpose
  MATLAB Function1 : MATLAB Function  TreatAsAtomicUnit=on
  Matrix Multiply : Product  Multiplication=Matrix(*)
  Matrix Multiply1 : Product  Multiplication=Matrix(*)
  Matrix Multiply2 : Product  Multiplication=Matrix(*)
  Max : MinMax  Function=max  Inputs=2
  Max1 : MinMax  Function=max  Inputs=2
  Max2 : MinMax  Function=max  Inputs=2
  Mux : Mux  Inputs=3
  Mux1 : Mux  Inputs=3
  Product{,1..5} (6 alike) : Product
  Reshape : Reshape  OutputDimensionality=Column vector (2-D)
  Reshape1 : Reshape  OutputDimensionality=Column vector (2-D)
  Scope : Scope
      settings: ActiveDisplayYMinimum=-2180.0732  ActiveDisplayYMaximum=4700.4941  DataLoggingVariableName=ScopeData15
  Scope1 : Scope
      settings: ActiveDisplayYMinimum=-2.3E-16  ActiveDisplayYMaximum=4.2E-16  DataLoggingVariableName=ScopeData16
  Scope2 : Scope
      settings: ActiveDisplayYMinimum=-8E-8  ActiveDisplayYMaximum=6.8E-7  DataLoggingVariableName=ScopeData17
  Selector : Selector  InputPortWidth=3  IndexOptions=Index vector (dialog)  Indices=2  OutputSizes=1
  Selector1 : Selector  InputPortWidth=3  IndexOptions=Index vector (dialog)  Indices=2  OutputSizes=1
  Selector2 : Selector  InputPortWidth=3  IndexOptions=Index vector (dialog)  Indices=2  OutputSizes=1
  Subsystem : Subsystem
  Subsystem1 : Subsystem
  Subsystem2 : Subsystem
  N_nose : Outport
  N_left : Outport  Port=2
  N_right : Outport  Port=3
  tag scope: N_left=global, N_nose=global, N_right=global, V_cg_b=global, V_left_g=global, V_left_y_g=global, V_nose_g=global, V_nose_y_g=global, V_right_g=global, V_right_y_g=global, omiga_b=global
  wires:
  [wx1] -> Mux/1
  [wz1] -> Scope1/1, Mux/3
  [wy1] -> Mux/2
  Mux/1 -> Reshape/1
  Reshape/1 -> [omiga_b]
  Constant2/1 -> Cross Product2/2
  Constant1/1 -> Cross Product1/2
  Constant/1 -> Cross Product/2
  [omiga_b] -> Cross Product1/1, Cross Product2/1, Cross Product/1
  [vy1] -> Scope2/1, Mux1/2
  [vx1] -> Mux1/1
  [vz1] -> Mux1/3
  Mux1/1 -> Reshape1/1
  Reshape1/1 -> [V_cg_b]
  Cross Product/1 -> Add/2
  Cross Product1/1 -> Add1/2
  Cross Product2/1 -> Add2/2
  [V_cg_b] -> Add/1, Add1/1, Add2/1
  MATLAB Function1/1(R_gb) -> Hermitian Transpose/1
  [gamma_eular] -> MATLAB Function1/1(gamma)
  Add1/1 -> Matrix Multiply1/2
  Add2/1 -> Matrix Multiply2/2
  Add/1 -> Matrix Multiply/2
  Hermitian Transpose/1 -> Matrix Multiply/1, Matrix Multiply1/1, Matrix Multiply2/1
  Matrix Multiply/1 -> [V_nose_g], Selector/1
  Matrix Multiply1/1 -> [V_left_g], Selector1/1
  Matrix Multiply2/1 -> [V_right_g], Selector2/1
  Selector2/1 -> Gain2/1, [V_right_y_g]
  Selector1/1 -> Gain1/1, [V_left_y_g]
  Selector/1 -> Scope/1, Gain/1, [V_nose_y_g]
  Product/1 -> Add3/2
  Product3/1 -> Add3/1
  Product1/1 -> Add4/2
  Product2/1 -> Add5/2
  Product4/1 -> Add4/1
  Product5/1 -> Add5/1
  Add4/1 -> Subsystem1/1(In1)
  Add5/1 -> Subsystem2/1(In1)
  delta_nose/1 -> Product3/2
  delta_left/1 -> Product4/2
  delta_right/1 -> Product5/2
  Gain/1 -> Product/2
  Gain1/1 -> Product1/2
  Gain2/1 -> Product2/2
  [theta_eular] -> MATLAB Function1/2(theta)
  [psi_eular] -> MATLAB Function1/3(psi)
  Constant3/1 -> Demux/1
  Demux/1 -> Product/1
  Demux/3 -> Product2/1
  Constant4/1 -> Demux1/1
  Demux1/1 -> Product3/1
  Demux1/2 -> Product4/1
  Demux1/3 -> Product5/1
  Add3/1 -> Subsystem/1(In1)
  Max/1 -> [N_nose], N_nose/1
  Subsystem1/1(N_left) -> Max1/2
  Max1/1 -> [N_left], N_left/1
  Subsystem/1(N_nose) -> Max/2
  Subsystem2/1(N_right) -> Max2/2
  Max2/1 -> [N_right], N_right/1
  Constant5/1 -> Max2/1, Max1/1, Max/1
  Demux/2 -> Product1/1

== system planmodel_m/6DOF-MODEL/动力学/起落架模型/纵向力 ==
  delta_s(H) : Inport
  u_brake : Inport  Port=2
  Subsystem : Subsystem
  Subsystem1 : Subsystem
  F_long_nose : Outport
  F_long_left : Outport  Port=2
  F_long_right : Outport  Port=3
  wires:
  delta_s(H)/1 -> Subsystem/1(delt-s(H))
  Subsystem/1(V_long_nose) -> Subsystem1/1(V_long_nose)
  Subsystem/2(V_long_left) -> Subsystem1/2(V_long_left)
  Subsystem/3(V_long_right) -> Subsystem1/3(V_long_right)
  u_brake/1 -> Subsystem1/4(u_brake)
  Subsystem1/1(F_long_nose) -> F_long_nose/1
  Subsystem1/2(F_long_left) -> F_long_left/1
  Subsystem1/3(F_long_right) -> F_long_right/1

== system planmodel_m/6DOF-MODEL/动力学/起落架模型/起落架三轮质心在地系下位置 ==
  Add : Sum
  Add1 : Sum
  Add2 : Sum
  Constant : Constant  Value=r_nose_b
  Constant1 : Constant  Value=r_left_b
  Constant2 : Constant  Value=r_right_b
  MATLAB Function1 : MATLAB Function  TreatAsAtomicUnit=on
  Matrix Multiply : Product  Multiplication=Matrix(*)
  Matrix Multiply1 : Product  Multiplication=Matrix(*)
  Matrix Multiply2 : Product  Multiplication=Matrix(*)
  Mux : Mux  Inputs=3
  Scope : Scope
      settings: ActiveDisplayYMinimum=0.16301  ActiveDisplayYMaximum=0.18017  DataLoggingVariableName=ScopeData9
  Scope1 : Scope
      settings: ActiveDisplayYMinimum=800.0265  ActiveDisplayYMaximum=1029.6474  DataLoggingVariableName=ScopeData18
  Scope2 : Scope
      settings: ActiveDisplayYMinimum=-3.8379  ActiveDisplayYMaximum=0.42644  DataLoggingVariableName=ScopeData19
  Selector : Selector  InputPortWidth=3  IndexOptions=Index vector (dialog)  Indices=2  OutputSizes=1
  Transpose : matrix_library/Transpose
  Nose_pos_g : Outport
  Left_pos_g : Outport  Port=2
  Right_pos_g : Outport  Port=3
  tag scope: Left_pos_g=global, Nose_position_g=global, Right_pos_g=global
  wires:
  Constant1/1 -> Matrix Multiply1/2
  Transpose/1 -> Matrix Multiply2/1, Matrix Multiply1/1, Matrix Multiply/1
  [psi_eular] -> MATLAB Function1/3(psi)
  [gamma_eular] -> Scope2/1, MATLAB Function1/1(gamma)
  Constant2/1 -> Matrix Multiply2/2
  Matrix Multiply1/1 -> Add1/2
  Constant/1 -> Matrix Multiply/2
  [theta_eular] -> MATLAB Function1/2(theta)
  MATLAB Function1/1(R_gb) -> Transpose/1
  Matrix Multiply/1 -> Add/2
  Matrix Multiply2/1 -> Add2/2
  [Z_positon] -> Mux/3
  [Y_positon] -> Scope1/1, Mux/2
  [X_positon] -> Mux/1
  Mux/1 -> Add/1, Add1/1, Add2/1
  Add/1 -> Selector/1, Nose_pos_g/1, [Nose_position_g]
  Add1/1 -> Left_pos_g/1, [Left_pos_g]
  Add2/1 -> Right_pos_g/1, [Right_pos_g]
  Selector/1 -> Scope/1

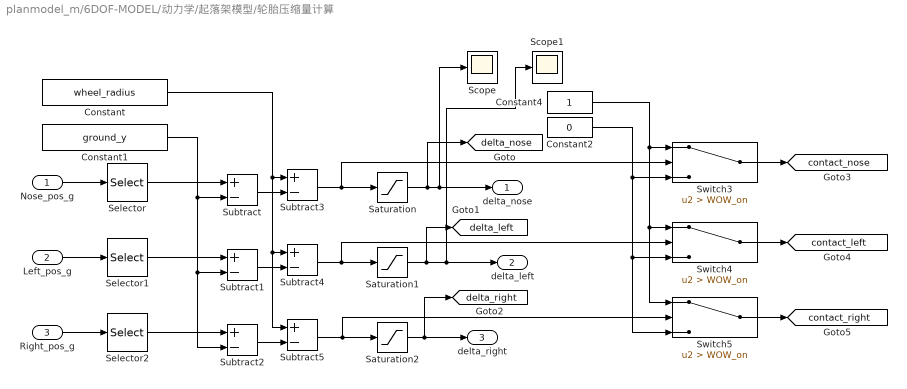
== system planmodel_m/6DOF-MODEL/动力学/起落架模型/轮胎压缩量计算 ==
  Nose_pos_g : Inport
  Left_pos_g : Inport  Port=2
  Right_pos_g : Inport  Port=3
  Constant : Constant  Value=wheel_radius
  Constant1 : Constant  Value=ground_y
  Constant2 : Constant  Value=0
  Constant4 : Constant
  Saturation : Saturate  UpperLimit=wheel_radius  LowerLimit=0
  Saturation1 : Saturate  UpperLimit=wheel_radius  LowerLimit=0
  Saturation2 : Saturate  UpperLimit=wheel_radius  LowerLimit=0
  Scope : Scope
      settings: ActiveDisplayYMinimum=-0.00105  ActiveDisplayYMaximum=0.00946  DataLoggingVariableName=ScopeData11
  Scope1 : Scope
      settings: ActiveDisplayYMinimum=-0.00123  ActiveDisplayYMaximum=0.01105  DataLoggingVariableName=ScopeData3
  Selector : Selector  InputPortWidth=3  IndexOptions=Index vector (dialog)  Indices=2  OutputSizes=1
  Selector1 : Selector  InputPortWidth=3  IndexOptions=Index vector (dialog)  Indices=2  OutputSizes=1
  Selector2 : Selector  InputPortWidth=3  IndexOptions=Index vector (dialog)  Indices=2  OutputSizes=1
  Subtract{,1..5} (6 alike) : Sum  Inputs=+-
  Switch3 : Switch  Criteria=u2 > Threshold  Threshold=WOW_on  SaturateOnIntegerOverflow=off  InputSameDT=off
  Switch4 : Switch  Criteria=u2 > Threshold  Threshold=WOW_on  SaturateOnIntegerOverflow=off  InputSameDT=off
  Switch5 : Switch  Criteria=u2 > Threshold  Threshold=WOW_on  SaturateOnIntegerOverflow=off  InputSameDT=off
  delta_nose : Outport
  delta_left : Outport  Port=2
  delta_right : Outport  Port=3
  tag scope: contact_left=global, contact_nose=global, contact_right=global, delta_left=global, delta_nose=global, delta_right=global
  wires:
  Nose_pos_g/1 -> Selector/1
  Left_pos_g/1 -> Selector1/1
  Right_pos_g/1 -> Selector2/1
  Selector/1 -> Subtract/1
  Selector1/1 -> Subtract1/1
  Selector2/1 -> Subtract2/1
  Constant1/1 -> Subtract/2, Subtract1/2, Subtract2/2
  Subtract/1 -> Subtract3/2
  Subtract1/1 -> Subtract4/2
  Subtract2/1 -> Subtract5/2
  Constant/1 -> Subtract5/1, Subtract4/1, Subtract3/1
  Saturation/1 -> Scope/1, delta_nose/1, [delta_nose]
  Saturation1/1 -> [delta_left], delta_left/1, Scope1/1
  Saturation2/1 -> [delta_right], delta_right/1
  Subtract3/1 -> Switch3/2, Saturation/1
  Subtract4/1 -> Switch4/2, Saturation1/1
  Subtract5/1 -> Switch5/2, Saturation2/1
  Constant2/1 -> Switch3/3, Switch5/3, Switch4/3
  Constant4/1 -> Switch5/1, Switch4/1, Switch3/1
  Switch3/1 -> [contact_nose]
  Switch5/1 -> [contact_right]
  Switch4/1 -> [contact_left]

== system planmodel_m/control/俯仰通道控制器/俯仰通道/伪攻角回路 ==
  wz : Inport
  Constant : Constant
  Integrator : Integrator  ExternalReset=either
  Product : Product
  Subsystem : Subsystem
  Sum : Sum  Inputs=|+-
  Sum3 : Sum  Inputs=|+-
  To Workspace : ToWorkspace  VariableName=a34  SaveFormat=Timeseries  SampleTime=-1
  alpha_c : Outport
  wires:
  wz/1 -> Sum/1
  Sum/1 -> Integrator/1
  Integrator/1 -> alpha_c/1, Product/2
  Product/1 -> Sum/2
  Subsystem/1(a34) -> Product/1, To Workspace/1
  Sum3/1 -> Integrator/2
  [no_contact] -> Sum3/2
  Constant/1 -> Sum3/1

== system planmodel_m/control/航向通道控制器/偏航通道/伪攻角回路 ==
  wy : Inport
  Constant1 : Constant
  Constant3 : Constant  Value=0
  Integrator : Integrator  ExternalReset=either
  Product : Product
  Subsystem : Subsystem
  Sum : Sum  Inputs=|+-
  Switch2 : Switch  Threshold=40  SaturateOnIntegerOverflow=off  InputSameDT=off
  beta_c : Outport
  wires:
  wy/1 -> Sum/1
  Sum/1 -> Integrator/1
  Integrator/1 -> beta_c/1, Product/2
  Product/1 -> Sum/2
  Subsystem/1(b) -> Product/1
  [Vg] -> Switch2/2
  Constant1/1 -> Switch2/1
  Constant3/1 -> Switch2/3
  Switch2/1 -> Integrator/2

== system planmodel_m/control/航向通道控制器1/偏航通道/伪攻角回路 ==
  wy : Inport
  Constant1 : Constant
  Constant3 : Constant  Value=0
  Integrator : Integrator  ExternalReset=either
  Product : Product
  Subsystem : Subsystem
  Sum : Sum  Inputs=|+-
  Switch2 : Switch  Threshold=40  SaturateOnIntegerOverflow=off  InputSameDT=off
  beta_c : Outport
  wires:
  wy/1 -> Sum/1
  Sum/1 -> Integrator/1
  Integrator/1 -> beta_c/1, Product/2
  Product/1 -> Sum/2
  Subsystem/1(b) -> Product/1
  [Vg] -> Switch2/2
  Constant1/1 -> Switch2/1
  Constant3/1 -> Switch2/3
  Switch2/1 -> Integrator/2

== system planmodel_m/6DOF-MODEL/动力学/起落架模型/三轮在地系下的力/摩擦圆限幅 ==
  N_nose : Inport
  N_left : Inport  Port=2
  N_right : Inport  Port=3
  F_long_nose : Inport  Port=4
  F_long_left : Inport  Port=5
  F_long_right : Inport  Port=6
  F_lat_nose : Inport  Port=7
  F_lat_left : Inport  Port=8
  F_lat_right : Inport  Port=9
  主轮摩擦圆限幅右 : MATLAB Function  TreatAsAtomicUnit=on
  主轮摩擦圆限幅左 : MATLAB Function  TreatAsAtomicUnit=on
  前轮摩擦圆限幅 : MATLAB Function  TreatAsAtomicUnit=on
  F_long_nose_out : Outport
  F_long_left_out : Outport  Port=2
  F_long_right_out : Outport  Port=3
  F_lat__nose_out : Outport  Port=4
  F_lat_left_out : Outport  Port=5
  F_lat_right_out : Outport  Port=6
  wires:
  前轮摩擦圆限幅/1(F_long_out) -> F_long_nose_out/1
  前轮摩擦圆限幅/2(F_lat_out) -> F_lat__nose_out/1
  主轮摩擦圆限幅左/2(F_lat_out) -> F_lat_left_out/1
  主轮摩擦圆限幅左/1(F_long_out) -> F_long_left_out/1
  主轮摩擦圆限幅右/2(F_lat_out) -> F_lat_right_out/1
  主轮摩擦圆限幅右/1(F_long_out) -> F_long_right_out/1
  N_nose/1 -> 前轮摩擦圆限幅/1(N)
  F_long_nose/1 -> 前轮摩擦圆限幅/2(F_long)
  F_lat_nose/1 -> 前轮摩擦圆限幅/3(F_lat)
  F_long_left/1 -> 主轮摩擦圆限幅左/2(F_long)
  N_left/1 -> 主轮摩擦圆限幅左/1(N)
  F_lat_right/1 -> 主轮摩擦圆限幅右/3(F_lat)
  F_lat_left/1 -> 主轮摩擦圆限幅左/3(F_lat)
  F_long_right/1 -> 主轮摩擦圆限幅右/2(F_long)
  N_right/1 -> 主轮摩擦圆限幅右/1(N)

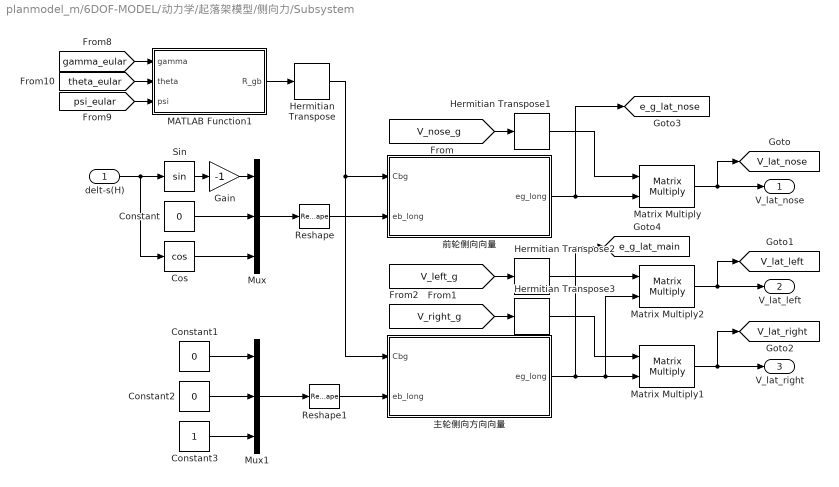
== system planmodel_m/6DOF-MODEL/动力学/起落架模型/侧向力/Subsystem ==
  delt-s(H) : Inport
  Constant : Constant  Value=0
  Constant1 : Constant  Value=0
  Constant2 : Constant  Value=0
  Constant3 : Constant
  Cos : Trigonometry  Operator=cos
  Gain : Gain  Gain=-1
  Hermitian Transpose{,1..3} (4 alike) : matrix_library/Hermitian Transpose
  MATLAB Function1 : MATLAB Function  TreatAsAtomicUnit=on
  Matrix Multiply : Product  Multiplication=Matrix(*)
  Matrix Multiply1 : Product  Multiplication=Matrix(*)
  Matrix Multiply2 : Product  Multiplication=Matrix(*)
  Mux : Mux  Inputs=3
  Mux1 : Mux  Inputs=3
  Reshape : Reshape  OutputDimensionality=Column vector (2-D)
  Reshape1 : Reshape  OutputDimensionality=Column vector (2-D)
  Sin : Trigonometry
  主轮侧向方向向量 : MATLAB Function  TreatAsAtomicUnit=on
  前轮侧向向量 : MATLAB Function  TreatAsAtomicUnit=on
  V_lat_nose : Outport
  V_lat_left : Outport  Port=2
  V_lat_right : Outport  Port=3
  tag scope: V_lat_left=global, V_lat_nose=global, V_lat_right=global, e_g_lat_main=global, e_g_lat_nose=global
  wires:
  MATLAB Function1/1(R_gb) -> Hermitian Transpose/1
  [gamma_eular] -> MATLAB Function1/1(gamma)
  Hermitian Transpose/1 -> 主轮侧向方向向量/1(Cbg), 前轮侧向向量/1(Cbg)
  Constant/1 -> Mux/2
  Mux/1 -> Reshape/1
  Constant1/1 -> Mux1/1
  Constant2/1 -> Mux1/2
  Constant3/1 -> Mux1/3
  Mux1/1 -> Reshape1/1
  [V_nose_g] -> Hermitian Transpose1/1
  前轮侧向向量/1(eg_long) -> [e_g_lat_nose], Matrix Multiply/2
  Hermitian Transpose1/1 -> Matrix Multiply/1
  [V_left_g] -> Hermitian Transpose2/1
  [V_right_g] -> Hermitian Transpose3/1
  主轮侧向方向向量/1(eg_long) -> Matrix Multiply2/2, Matrix Multiply1/2, [e_g_lat_main]
  Hermitian Transpose3/1 -> Matrix Multiply1/1
  Hermitian Transpose2/1 -> Matrix Multiply2/1
  Matrix Multiply/1 -> V_lat_nose/1, [V_lat_nose]
  Matrix Multiply2/1 -> V_lat_left/1, [V_lat_left]
  Matrix Multiply1/1 -> V_lat_right/1, [V_lat_right]
  Cos/1 -> Mux/3
  Sin/1 -> Gain/1
  Gain/1 -> Mux/1
  delt-s(H)/1 -> Sin/1, Cos/1
  [theta_eular] -> MATLAB Function1/2(theta)
  [psi_eular] -> MATLAB Function1/3(psi)
  Reshape/1 -> 前轮侧向向量/2(eb_long)
  Reshape1/1 -> 主轮侧向方向向量/2(eb_long)

== system planmodel_m/6DOF-MODEL/动力学/起落架模型/侧向力/Subsystem1 ==
  In1 : Inport
  Constant5 : Constant  Value=0
  Switch : Switch  Criteria=u2 > Threshold  SaturateOnIntegerOverflow=off  InputSameDT=off
  F_lat_left : Outport
  wires:
  In1/1 -> Switch/1
  Constant5/1 -> Switch/3
  Switch/1 -> F_lat_left/1
  [contact_left] -> Switch/2

== system planmodel_m/6DOF-MODEL/动力学/起落架模型/侧向力/Subsystem2 ==
  In1 : Inport
  Constant5 : Constant  Value=0
  Switch : Switch  Criteria=u2 > Threshold  SaturateOnIntegerOverflow=off  InputSameDT=off
  F_lat_nose : Outport
  wires:
  In1/1 -> Switch/1
  Constant5/1 -> Switch/3
  Switch/1 -> F_lat_nose/1
  [contact_nose] -> Switch/2

== system planmodel_m/6DOF-MODEL/动力学/起落架模型/侧向力/Subsystem3 ==
  In1 : Inport
  Constant5 : Constant  Value=0
  Switch : Switch  Criteria=u2 > Threshold  SaturateOnIntegerOverflow=off  InputSameDT=off
  F_lat_right : Outport
  wires:
  [contact_right] -> Switch/2
  Switch/1 -> F_lat_right/1
  Constant5/1 -> Switch/3
  In1/1 -> Switch/1

== system planmodel_m/6DOF-MODEL/动力学/起落架模型/法向支反力/Subsystem ==
  In1 : Inport
  Constant5 : Constant  Value=0
  Switch : Switch  Criteria=u2 > Threshold  SaturateOnIntegerOverflow=off  InputSameDT=off
  N_nose : Outport
  wires:
  In1/1 -> Switch/1
  Constant5/1 -> Switch/3
  Switch/1 -> N_nose/1
  [contact_nose] -> Switch/2

== system planmodel_m/6DOF-MODEL/动力学/起落架模型/法向支反力/Subsystem1 ==
  In1 : Inport
  Constant5 : Constant  Value=0
  Switch : Switch  Criteria=u2 > Threshold  SaturateOnIntegerOverflow=off  InputSameDT=off
  N_left : Outport
  wires:
  [contact_left] -> Switch/2
  Switch/1 -> N_left/1
  Constant5/1 -> Switch/3
  In1/1 -> Switch/1

== system planmodel_m/6DOF-MODEL/动力学/起落架模型/法向支反力/Subsystem2 ==
  In1 : Inport
  Constant5 : Constant  Value=0
  Switch : Switch  Criteria=u2 > Threshold  SaturateOnIntegerOverflow=off  InputSameDT=off
  N_right : Outport
  wires:
  In1/1 -> Switch/1
  Constant5/1 -> Switch/3
  Switch/1 -> N_right/1
  [contact_right] -> Switch/2

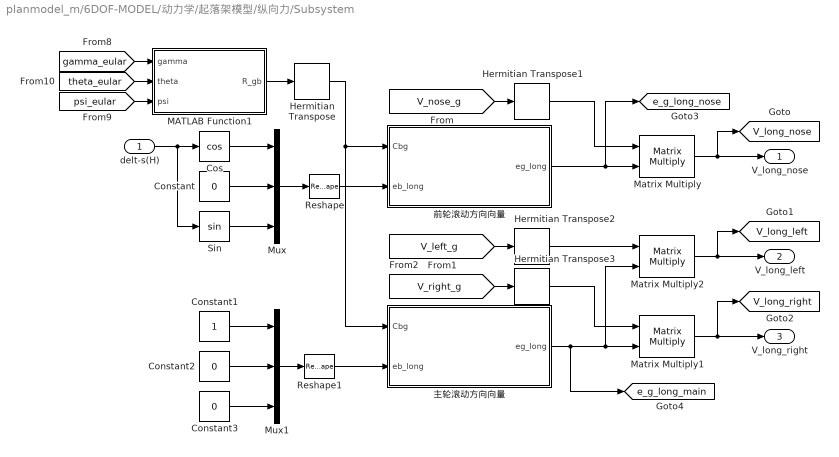
== system planmodel_m/6DOF-MODEL/动力学/起落架模型/纵向力/Subsystem ==
  delt-s(H) : Inport
  Constant : Constant  Value=0
  Constant1 : Constant
  Constant2 : Constant  Value=0
  Constant3 : Constant  Value=0
  Cos : Trigonometry  Operator=cos
  Hermitian Transpose{,1..3} (4 alike) : matrix_library/Hermitian Transpose
  MATLAB Function1 : MATLAB Function  TreatAsAtomicUnit=on
  Matrix Multiply : Product  Multiplication=Matrix(*)
  Matrix Multiply1 : Product  Multiplication=Matrix(*)
  Matrix Multiply2 : Product  Multiplication=Matrix(*)
  Mux : Mux  Inputs=3
  Mux1 : Mux  Inputs=3
  Reshape : Reshape  OutputDimensionality=Column vector (2-D)
  Reshape1 : Reshape  OutputDimensionality=Column vector (2-D)
  Sin : Trigonometry
  主轮滚动方向向量 : MATLAB Function  TreatAsAtomicUnit=on
  前轮滚动方向向量 : MATLAB Function  TreatAsAtomicUnit=on
  V_long_nose : Outport
  V_long_left : Outport  Port=2
  V_long_right : Outport  Port=3
  tag scope: V_long_left=global, V_long_nose=global, V_long_right=global, e_g_long_main=global, e_g_long_nose=global
  wires:
  MATLAB Function1/1(R_gb) -> Hermitian Transpose/1
  [gamma_eular] -> MATLAB Function1/1(gamma)
  Hermitian Transpose/1 -> 主轮滚动方向向量/1(Cbg), 前轮滚动方向向量/1(Cbg)
  delt-s(H)/1 -> Cos/1, Sin/1
  Cos/1 -> Mux/1
  Constant/1 -> Mux/2
  Sin/1 -> Mux/3
  Mux/1 -> Reshape/1
  Constant1/1 -> Mux1/1
  Constant2/1 -> Mux1/2
  Constant3/1 -> Mux1/3
  Mux1/1 -> Reshape1/1
  [V_nose_g] -> Hermitian Transpose1/1
  前轮滚动方向向量/1(eg_long) -> [e_g_long_nose], Matrix Multiply/2
  Hermitian Transpose1/1 -> Matrix Multiply/1
  [V_left_g] -> Hermitian Transpose2/1
  [V_right_g] -> Hermitian Transpose3/1
  主轮滚动方向向量/1(eg_long) -> Matrix Multiply1/2, Matrix Multiply2/2, [e_g_long_main]
  Hermitian Transpose3/1 -> Matrix Multiply1/1
  Hermitian Transpose2/1 -> Matrix Multiply2/1
  Matrix Multiply/1 -> V_long_nose/1, [V_long_nose]
  Matrix Multiply2/1 -> V_long_left/1, [V_long_left]
  Matrix Multiply1/1 -> V_long_right/1, [V_long_right]
  [theta_eular] -> MATLAB Function1/2(theta)
  [psi_eular] -> MATLAB Function1/3(psi)
  Reshape/1 -> 前轮滚动方向向量/2(eb_long)
  Reshape1/1 -> 主轮滚动方向向量/2(eb_long)
